simulink model "Depth_Plane_AUV_NN_EKF"  (R2021a)
settings: Solver=VariableStepAuto  StartTime=0.0  StopTime=10.0  RelTol=1e-3
libraries: pid_lib x1
settings Model: Creator=7385281  LastModifiedBy=7385281
settings DataIOCC: ReturnWorkspaceOutputs=off

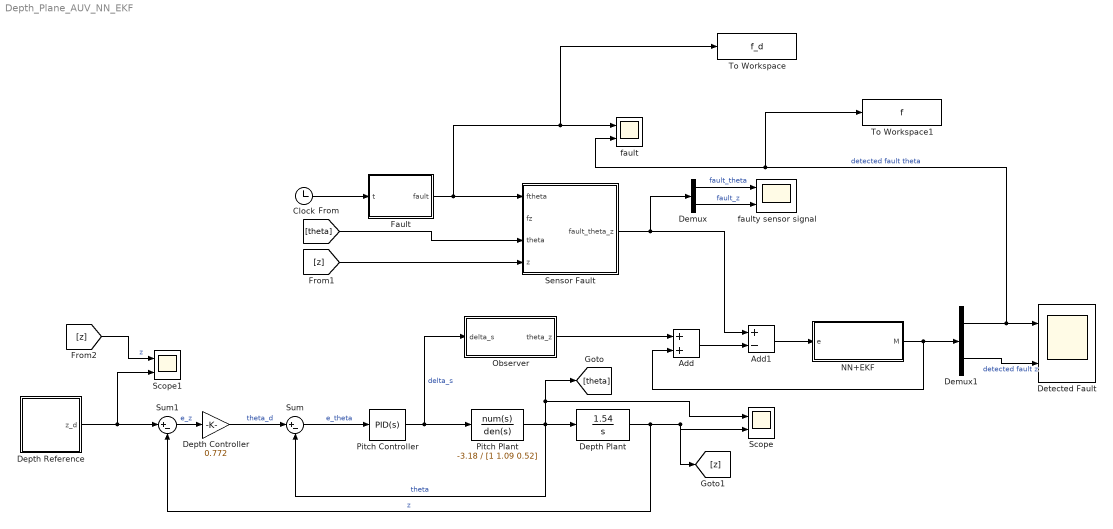
== system Depth_Plane_AUV_NN_EKF ==
  Add : Sum
  Add1 : Sum  Inputs=+-
  Clock : Clock
  Demux : Demux  Outputs=2
  Demux1 : Demux  Outputs=2
  Depth Controller : Gain  Gain=0.772
  Depth Plant : TransferFcn  Numerator=1.54  Denominator=[1 0]
  Depth Reference : Subsystem
  Detected Fault : Scope  NumInputPorts=2
  Fault : MATLAB Function  TreatAsAtomicUnit=on
  NN+EKF : Subsystem
  Observer : Subsystem
  Pitch Controller : pid_lib/PID Controller  Controller=PID  Form=Parallel  TimeDomain=Continuous-time  UseExternalTs=off  SampleTime=-1  IntegratorMethod=Forward Euler  FilterMethod=Forward Euler  ControllerParametersSource=internal  P=-10.43  I=0  D=0.21*-10.43  UseFilter=on  N=100  TunerSelectOption=Transfer Function Based (PID Tuner App)  InitialConditionSource=internal  InitialConditionForIntegrator=0  InitialConditionForFilter=0  DifferentiatorICPrevScaledInput=0  ExternalReset=none  TrackingMode=off  Kt=1  LimitOutput=off  SatLimitsSource=internal  UpperSaturationLimit=inf  LowerSaturationLimit=-inf  LinearizeAsGain=on  AntiWindupMode=none  Kb=1  POutMin=[]  POutMax=[]  IOutMin=[]  IOutMax=[]  DOutMin=[]  DOutMax=[]  NOutMin=[]  NOutMax=[]  SumOutMin=[]  SumOutMax=[]  SaturationOutMin=[]  SaturationOutMax=[]  PParamMin=[]  PParamMax=[]  IParamMin=[]  IParamMax=[]  DParamMin=[]  DParamMax=[]  NParamMin=[]  NParamMax=[]  KbParamMin=[]  KbParamMax=[]  KtParamMin=[]  KtParamMax=[]  KbOutMin=[]  KbOutMax=[]  KtOutMin=[]  KtOutMax=[]  IntegratorOutMin=[]  IntegratorOutMax=[]  FilterOutMin=[]  FilterOutMax=[]  SumI1OutMin=[]  SumI1OutMax=[]  SumI2OutMin=[]  SumI2OutMax=[]  SumI3OutMin=[]  SumI3OutMax=[]  SumI4OutMin=[]  SumI4OutMax=[]  SumDOutMin=[]  SumDOutMax=[]  DifferentiatorOutMin=[]  DifferentiatorOutMax=[]  FilterDiffOutCoefMin=[]  FilterDiffOutCoefMax=[]  ReciprocalOutMin=[]  ReciprocalOutMax=[]  SumDenOutMin=[]  SumDenOutMax=[]  SumNumOutMin=[]  SumNumOutMax=[]  DivideOutMin=[]  DivideOutMax=[]  UdiffTsProdOutMin=[]  UdiffTsProdOutMax=[]  NTsProdOutMin=[]  NTsProdOutMax=[]  UintegralTsProdOutMin=[]  UintegralTsProdOutMax=[]  UngainTsProdOutMin=[]  UngainTsProdOutMax=[]  IntegratorContinuousStateAttributes=''  IntegratorStateMustResolveToSignalObject=off  IntegratorRTWStateStorageClass=Auto  FilterContinuousStateAttributes=''  FilterStateMustResolveToSignalObject=off  FilterRTWStateStorageClass=Auto  ParallelPVariant=InternalParameters  IdealPVariant=Disabled  IVariant=InternalParameters  DVariant=InternalParameters  IntegratorVariant=Continuous  SatVariant=Disabled  AWVariant=Passthrough  PCopyVariant=Disabled  TRVariant=Disabled  FdbkBlocksVariant=Forward  IdealPFdbkVariant=Disabled  SatFdbkVariant=Disabled  DerivativeFilterVariant=ContFilter  NVariant=InternalParameters  NCopyVariant=Disabled  FilterICVariant=InternalICsFilter  IntegratorICVariant=InternalICs  ExternalResetVariant=Disabled  TRSumVariant=Passthrough  SumFdbkVariant=Disabled  SumVariant=Sum_PID  TsampFilterVariant=InternalTs  TsampNgainVariant=Passthrough  TsampIntegralVariant=Passthrough  ExternalSaturationOutDataTypeStr=Inherit: Same as second input
  Pitch Plant : TransferFcn  Numerator=-3.18  Denominator=[1 1.09 0.52]
  Scope : Scope  NumInputPorts=2
  Scope1 : Scope  NumInputPorts=2
  Sensor Fault : MATLAB Function  TreatAsAtomicUnit=on
  Sum : Sum  Inputs=|+-
  Sum1 : Sum  Inputs=|+-
  To Workspace : ToWorkspace  VariableName=f_d  SampleTime=-1
  To Workspace1 : ToWorkspace  VariableName=f  SampleTime=-1
  fault : Scope  NumInputPorts=2
  faulty sensor signal : Scope  NumInputPorts=2
  wires:
  Sum/1 -> Pitch Controller/1  "e_theta"
  Pitch Controller/1 -> Observer/1(delta_s), Pitch Plant/1  "delta_s"
  Pitch Plant/1 -> Scope/1, [theta], Depth Plant/1, Sum/2  "theta"
  Depth Controller/1 -> Sum/1  "theta_d"
  Sum1/1 -> Depth Controller/1  "e_z"
  Depth Plant/1 -> [z], Scope/2, Sum1/2  "z"
  Add/1 -> Add1/2
  Add1/1 -> NN+EKF/1(e)
  NN+EKF/1(M) -> Add/2, Demux1/1
  Clock/1 -> Fault/1(t)
  Sensor Fault/1(fault_theta_z) -> Demux/1, Add1/1
  Fault/1(fault) -> To Workspace/1, fault/1, Sensor Fault/1(ftheta)
  [z] -> Sensor Fault/4(z)
  [theta] -> Sensor Fault/3(theta)
  Observer/1(theta_z) -> Add/1
  Demux/1 -> faulty sensor signal/1  "fault_theta"
  Demux/2 -> faulty sensor signal/2  "fault_z"
  Demux1/1 -> To Workspace1/1, fault/2, Detected Fault/1  "detected fault theta"
  Demux1/2 -> Detected Fault/2  "detected fault z"
  [z] -> Scope1/1  "z"
  Depth Reference/1(z_d) -> Scope1/2, Sum1/1

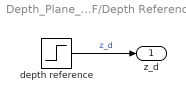
== system Depth_Plane_AUV_NN_EKF/Depth Reference ==
  depth reference : Step  Time=0  After=10  SampleTime=0
  z_d : Outport
  wires:
  depth reference/1 -> z_d/1  "z_d"

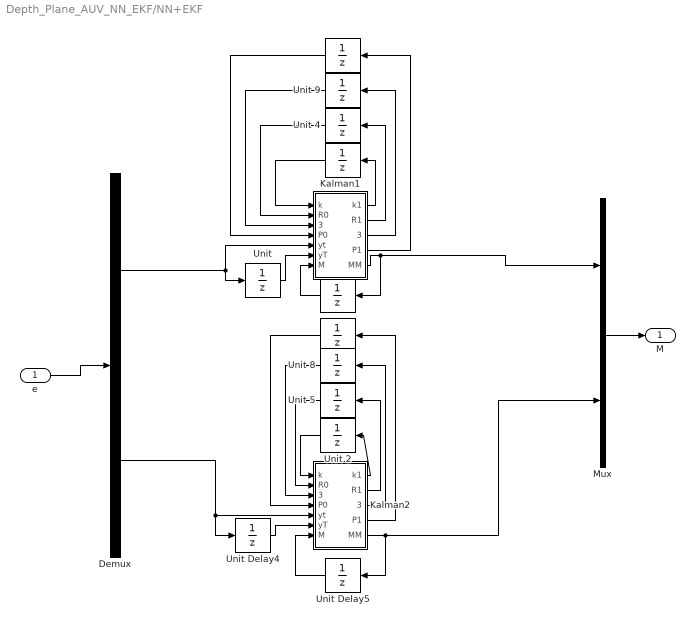
== system Depth_Plane_AUV_NN_EKF/NN+EKF ==
  e : Inport
  " " : UnitDelay  InitialCondition=1  SampleTime=-1  HasFrameUpgradeWarning=on
  "  " : UnitDelay  InitialCondition=5*eye(3)  SampleTime=-1  HasFrameUpgradeWarning=on
  "   " : UnitDelay  InitialCondition=5*eye(3)  SampleTime=-1  HasFrameUpgradeWarning=on
  "      " : UnitDelay  InitialCondition=.01  SampleTime=-1  HasFrameUpgradeWarning=on
  Demux : Demux  Outputs=2
  Kalman1 : MATLAB Function  TreatAsAtomicUnit=on
  Kalman2 : MATLAB Function  TreatAsAtomicUnit=on
  Mux : Mux  Inputs=2
  "Unit " : UnitDelay  SampleTime=-1  HasFrameUpgradeWarning=on
  Unit 2 : UnitDelay  InitialCondition=1  SampleTime=-1  HasFrameUpgradeWarning=on
  Unit 4 : UnitDelay  InitialCondition=.00002  SampleTime=-1  HasFrameUpgradeWarning=on
  Unit 5 : UnitDelay  InitialCondition=.00002  SampleTime=-1  HasFrameUpgradeWarning=on
  Unit 8 : UnitDelay  InitialCondition=[1;.5;.5]  SampleTime=-1  HasFrameUpgradeWarning=on
  Unit 9 : UnitDelay  InitialCondition=[1;.5;.5]  SampleTime=-1  HasFrameUpgradeWarning=on
  Unit Delay4 : UnitDelay  SampleTime=-1  HasFrameUpgradeWarning=on
  Unit Delay5 : UnitDelay  InitialCondition=.01  SampleTime=-1  HasFrameUpgradeWarning=on
  M : Outport
  wires:
  "      "/1 -> Kalman1/7(M)
  Kalman1/2(R1) -> Unit 4/1
  Kalman1/5(MM) -> Mux/1, "      "/1
  "Unit "/1 -> Kalman1/6(yT)
  Demux/1 -> "Unit "/1, Kalman1/5(yt)
  Kalman1/4(P1) -> "  "/1
  Unit 2/1 -> Kalman2/1(k)
  Kalman1/1(k1) -> " "/1
  Unit 8/1 -> Kalman2/3(teta0)
  Kalman2/4(P1) -> "   "/1
  Kalman2/2(R1) -> Unit 5/1
  " "/1 -> Kalman1/1(k)
  "   "/1 -> Kalman2/4(P0)
  Unit Delay4/1 -> Kalman2/6(yT)
  Demux/2 -> Kalman2/5(yt), Unit Delay4/1
  Unit Delay5/1 -> Kalman2/7(M)
  Unit 5/1 -> Kalman2/2(R0)
  Kalman2/3(teta1) -> Unit 8/1
  Unit 9/1 -> Kalman1/3(teta0)
  Kalman1/3(teta1) -> Unit 9/1
  Kalman2/5(MM) -> Mux/2, Unit Delay5/1
  Kalman2/1(k1) -> Unit 2/1
  "  "/1 -> Kalman1/4(P0)
  Unit 4/1 -> Kalman1/2(R0)
  e/1 -> Demux/1
  Mux/1 -> M/1

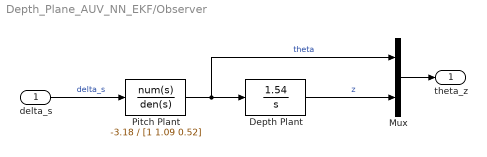
== system Depth_Plane_AUV_NN_EKF/Observer ==
  delta_s : Inport
  Depth Plant : TransferFcn  Numerator=1.54  Denominator=[1 0]
  Mux : Mux  Inputs=2
  Pitch Plant : TransferFcn  Numerator=-3.18  Denominator=[1 1.09 0.52]
  theta_z : Outport
  wires:
  Pitch Plant/1 -> Mux/1, Depth Plant/1  "theta"
  delta_s/1 -> Pitch Plant/1  "delta_s"
  Depth Plant/1 -> Mux/2  "z"
  Mux/1 -> theta_z/1

== matlab function Depth_Plane_AUV_NN_EKF/Sensor Fault ==
  data: ftheta input; fault_theta_z output; fz input; theta input; z input
function fault_theta_z = fcn(ftheta,fz,theta,z)
% This function creates the faulty signal from the sensor
fault_theta_z = [theta; z]+[ftheta; fz]+[0.0006; 0.000001];
end

== matlab function Depth_Plane_AUV_NN_EKF/Fault ==
  data: t input; fault output
function fault = fcn(t)
% This function creates the fault
t0=5;
omega=0.01;
if t<=t0
    fault=0;
else
    fault=1-exp(-omega*(t-t0));
end

== matlab function Depth_Plane_AUV_NN_EKF/NN+EKF/Kalman1 ==
  data: k1 output; R1 output; teta1 output; P1 output; k input; R0 input; teta0 input; P0 input; MM output; yt input; yT input; M input
function [k1,R1,teta1,P1,MM]  = fcn(k,R0,teta0,P0,yt,yT,M)
eta=1.5;
Z=teta0(2)*M+teta0(3)*yT;
sigma=(1-exp(-Z))/(1+exp(-Z));
H=[sigma;teta0(1)*M*0.5*(1-sigma^2);teta0(1)*yT*0.5*(1-sigma^2)];
R1=R0+(yt^2-R0)/k;
K=P0*H*(((H'*P0*H)+R1)^(-1));
teta1=teta0+eta*K*(yt);
n=teta1(2)*M+teta1(3)*yT;
MM=teta1(1)*((1-exp(-n))/(1+exp(-n)));
P1=P0-K*H'*P0;
k1=k+1;

== matlab function Depth_Plane_AUV_NN_EKF/NN+EKF/Kalman2 ==
  data: k1 output; R1 output; teta1 output; P1 output; k input; R0 input; teta0 input; P0 input; MM output; yt input; yT input; M input
function [k1,R1,teta1,P1,MM]  = fcn(k,R0,teta0,P0,yt,yT,M)
eta=1;
Z=teta0(2)*M+teta0(3)*yT;
sigma=(1-exp(-Z))/(1+exp(-Z));
H=[sigma;teta0(1)*M*.5*(1-sigma^2);teta0(1)*yT*0.5*(1-sigma^2)];
R1=R0+(yt^2-R0)/k;
K=P0*H*(((H'*P0*H)+R1)^(-1));
teta1=teta0+eta*K*(yt);
n=teta1(2)*M+teta1(3)*yT;
MM=teta1(1)*((1-exp(-n))/(1+exp(-n)));
P1=P0-K*H'*P0;
k1=k+1;
